simulink model "second_order_diff_simple"  (R2022a)
settings: Solver=VariableStepAuto  StartTime=0.0  StopTime=10.0  RelTol=1e-3
settings Model: Creator=Home computer  LastModifiedBy=Home computer

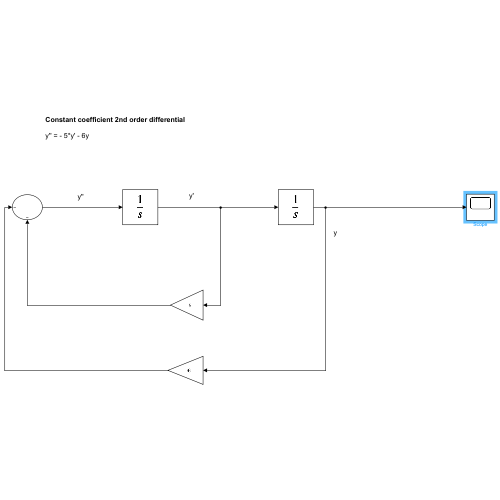
[thumbnail: Simulink's stored preview of the top-level diagram]
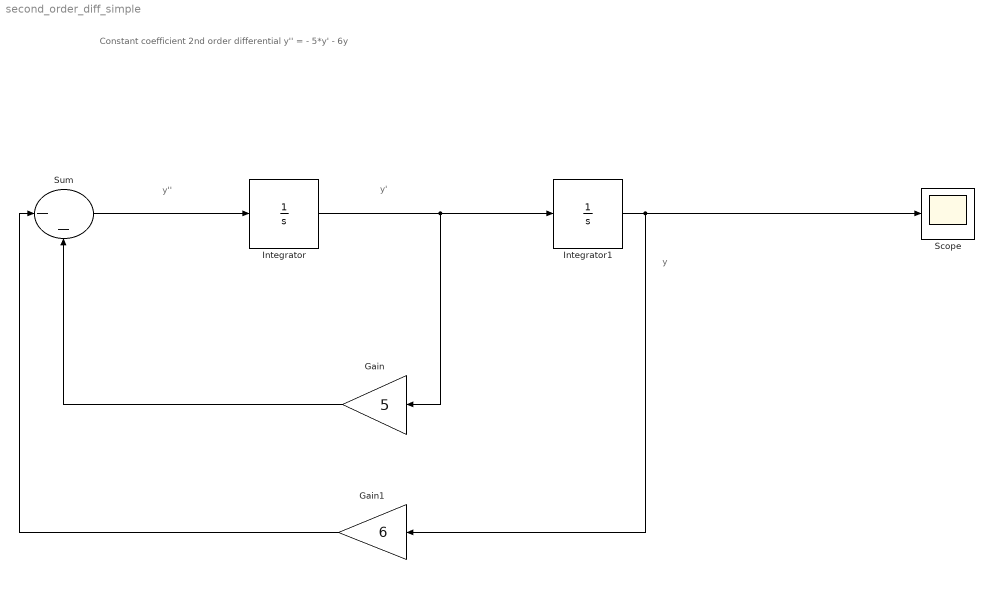
== system second_order_diff_simple ==
  note: Constant coefficient 2nd order differential
      |
      | y'' = - 5*y' - 6y
  note: y''
  note: y
  note: y'
  Gain : Gain  Gain=5
  Gain1 : Gain  Gain=6
  Integrator : Integrator  InitialCondition=1
  Integrator1 : Integrator
  Scope : Scope
  Sum : Sum  Inputs=|--
  wires:
  Integrator/1 -> Gain/1, Integrator1/1
  Gain/1 -> Sum/2
  Integrator1/1 -> Gain1/1, Scope/1
  Gain1/1 -> Sum/1
  Sum/1 -> Integrator/1
